simulink model "equalizer_model_deluxe"  (R2014a)
settings: Solver=ode45  StartTime=0.0  StopTime=inf  RelTol=1e-3
libraries: dsparch4 x15, dspmtrx3 x2, dspvision x1, dspobslib x1, dspsrcs4 x1, dspsnks4 x1, dspsigops x1
settings Model: Creator=salvat06  LastModifiedBy=salvat06
settings DebuggingCC: MergeDetectMultiDrivingBlocksExec=error

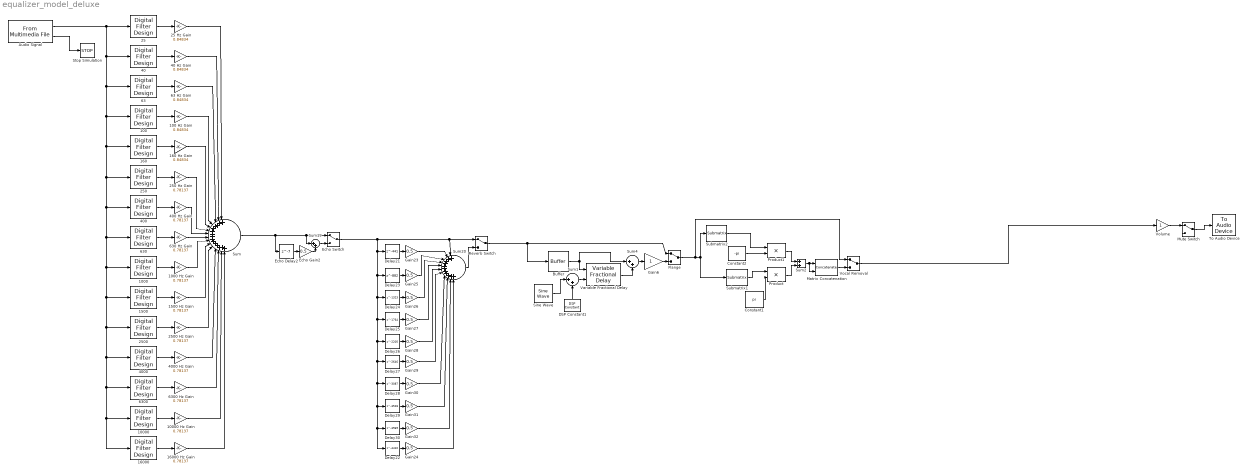
== system equalizer_model_deluxe ==
  {63,100,160,250,400,630,1000,1500,2500,4000,6300,10000,16000} (13 alike) : dsparch4/Digital Filter Design  mwdsp_browser_bugfix_var=off
  100 Hz Gain : Gain  Gain=0.84834
  1000 Hz Gain : Gain  Gain=0.78137
  10000 Hz Gain : Gain  Gain=0.78137
  1500 Hz Gain : Gain  Gain=0.78137
  160 Hz Gain : Gain  Gain=0.84834
  16000 Hz Gain : Gain  Gain=0.78137
  "25 " : dsparch4/Digital Filter Design  mwdsp_browser_bugfix_var=off
  25 Hz Gain : Gain  Gain=0.84834
  250 Hz Gain : Gain  Gain=0.78137
  2500 Hz Gain : Gain  Gain=0.78137
  "40 " : dsparch4/Digital Filter Design  mwdsp_browser_bugfix_var=off
  40 Hz Gain : Gain  Gain=0.84834
  400 Hz Gain : Gain  Gain=0.78137
  4000 Hz Gain : Gain  Gain=0.78137
  63 Hz Gain : Gain  Gain=0.84834
  630 Hz Gain : Gain  Gain=0.78137
  6300 Hz Gain : Gain  Gain=0.78137
  Audio Signal : dspvision/From Multimedia File  inputFilename=\\rowanads.rowan.edu\home\salvat06\documents\A-DSP, Round 2\McCall\James Music Selection\Iron Jaw Gulch.wav  loop=on  numPlays=1  outputStreams=Audio only  videoDataType=single  audioDataType=double  inheritSampleTime=on  userDefinedSampleTime=1/30  noAudioOutput=off  isIntensityVideo=off  fourcc=RGB  colorVideoFormat=Separate color signals  outputEOF=on  dataOrg=Column-major  audioFrameSize=256  computeAudioFrameSize=off  outSamplingMode=Frame based
  Buffer : Buffer  N=256  ic=100
  Constant1 : Constant  Value=pi
  Constant2 : Constant  Value=-pi
  DSP Constant1 : dspobslib/DSP Constant  Value=30  SampleMode=Discrete  discreteOutput=Sample-based (interpret vectors as 1-D)  continuousOutput=Sample-based (interpret vectors as 1-D)  sampTime=256/44100  framePeriod=256/44100  dataType=Inherit from 'Constant value'  isSigned=on  wordLen=16  udDataType=sfix(16)  fracBitsMode=Best precision  numFracBits=15  InterpretAs1D=on  Ts=256/44100  FramebasedOutput=off
  Delay21 : Delay  DelayLength=441  InitialCondition=0  InputProcessing=Inherited
  Delay22 : Delay  DelayLength=4410  InitialCondition=0  InputProcessing=Inherited
  Delay23 : Delay  DelayLength=882  InitialCondition=0  InputProcessing=Inherited
  Delay24 : Delay  DelayLength=1323  InitialCondition=0  InputProcessing=Inherited
  Delay25 : Delay  DelayLength=1764  InitialCondition=0  InputProcessing=Inherited
  Delay26 : Delay  DelayLength=2205  InitialCondition=0  InputProcessing=Inherited
  Delay27 : Delay  DelayLength=2646  InitialCondition=0  InputProcessing=Inherited
  Delay28 : Delay  DelayLength=3087  InitialCondition=0  InputProcessing=Inherited
  Delay29 : Delay  DelayLength=3528  InitialCondition=0  InputProcessing=Inherited
  Delay30 : Delay  DelayLength=3969  InitialCondition=0  InputProcessing=Inherited
  Echo Gain2 : Gain  Gain=0.5
  Echo Delay2 : Delay  DelayLength=7  InitialCondition=0  InputProcessing=Inherited
  Echo Switch : ManualSwitch
  Flange : ManualSwitch
  Gain{23..32} (10 alike) : Gain  Gain=0.5
  Gain6 : Gain  SaturateOnIntegerOverflow=on  OutDataTypeStr=Inherit: Same as input  ParamDataTypeStr=Inherit: Same as input
  Matrix Concatenation : Concatenate  Mode=Multidimensional array  ConcatenateDimension=2
  Mute Switch : ManualSwitch
  Product : Product  SaturateOnIntegerOverflow=on  OutDataTypeStr=Inherit: Same as first input
  Product1 : Product  SaturateOnIntegerOverflow=on  OutDataTypeStr=Inherit: Same as first input
  Reverb Switch : ManualSwitch
  Sine Wave : dspsrcs4/Sine Wave  Amplitude=30  Frequency=1/3.934 * 1.5  Phase=[-pi/4 pi/4]  SampleMode=Discrete  OutComplex=Real  CompMethod=Trigonometric fcn  TableSize=Speed  SampleTime=1/44100  SamplesPerFrame=256  ResetState=Restart at time zero  dataType=double  wordLen=16  udDataType=sfix(16)  fracBitsMode=User-defined  numFracBits=14  OutDataTypeStr=double  LastOutDataTypeStr=double
  Stop Simulation : Stop
  Submatrix1 : dspmtrx3/Submatrix  RowSpan=Range of rows  RowStartMode=First  RowStartIndex=1  RowEndMode=Last  RowEndIndex=1  ColSpan=One column  ColStartMode=Last  ColStartIndex=1  ColEndMode=Last  ColEndIndex=1
  Submatrix2 : dspmtrx3/Submatrix  RowSpan=Range of rows  RowStartMode=First  RowStartIndex=1  RowEndMode=Last  RowEndIndex=1  ColSpan=One column  ColStartMode=First  ColStartIndex=1  ColEndMode=Last  ColEndIndex=1
  Sum : Sum  Inputs=|+++++++++++++++  AccumDataTypeStr=double  OutDataTypeStr=double
  Sum1 : Sum  Inputs=|++  SaturateOnIntegerOverflow=on  InputSameDT=on  OutDataTypeStr=Inherit: Same as first input
  Sum19 : Sum  Inputs=|++
  Sum2 : Sum  SaturateOnIntegerOverflow=on
  Sum20 : Sum  Inputs=|+++++++++++
  Sum4 : Sum  Inputs=|++  SaturateOnIntegerOverflow=on  InputSameDT=on  OutDataTypeStr=Inherit: Same as first input
  To Audio Device : dspsnks4/To Audio Device  deviceName=Default  inheritSampleRate=off  sampleRate=44100  deviceDatatype=Determine from input data type  autoBufferSize=on  bufferSize=4096  queueDuration=1.0  defaultOutputChannelMapping=on  outputChannelMapping=1:2
  Variable Fractional Delay : dspsigops/Variable Fractional Delay  mode=OBSOLETE  modeActive=FIR  dmax=44100*10e-3  InputProcessing=Inherited (this choice will be removed - see release notes)  L=8  FarrowL=4  R=10  alpha=0.5  ic=0  fallbackFIR=Switch to linear interpolation if kernel cannot be centered  fallbackFarrow=Clip to the minimum value necessary for centered kernel  noDFT=off  roundingMode=Zero  overflowMode=off
  Vocal Removal : ManualSwitch
  Volume : Gain  Tag=Volume
  wires:
  "25 "/1 -> 25 Hz Gain/1
  "40 "/1 -> 40 Hz Gain/1
  63/1 -> 63 Hz Gain/1
  100/1 -> 100 Hz Gain/1
  160/1 -> 160 Hz Gain/1
  250/1 -> 250 Hz Gain/1
  400/1 -> 400 Hz Gain/1
  630/1 -> 630 Hz Gain/1
  1000/1 -> 1000 Hz Gain/1
  1500/1 -> 1500 Hz Gain/1
  2500/1 -> 2500 Hz Gain/1
  4000/1 -> 4000 Hz Gain/1
  6300/1 -> 6300 Hz Gain/1
  10000/1 -> 10000 Hz Gain/1
  16000/1 -> 16000 Hz Gain/1
  Audio Signal/2 -> Stop Simulation/1
  Vocal Removal/1 -> Volume/1
  Audio Signal/1 -> "25 "/1, "40 "/1, 63/1, 100/1, 160/1, 250/1, 400/1, 630/1, 1000/1, 1500/1, 4000/1, 6300/1, 10000/1, 16000/1, 2500/1
  25 Hz Gain/1 -> Sum/1
  40 Hz Gain/1 -> Sum/2
  63 Hz Gain/1 -> Sum/3
  100 Hz Gain/1 -> Sum/4
  250 Hz Gain/1 -> Sum/6
  160 Hz Gain/1 -> Sum/5
  400 Hz Gain/1 -> Sum/7
  630 Hz Gain/1 -> Sum/8
  1000 Hz Gain/1 -> Sum/9
  1500 Hz Gain/1 -> Sum/10
  2500 Hz Gain/1 -> Sum/11
  4000 Hz Gain/1 -> Sum/12
  6300 Hz Gain/1 -> Sum/13
  10000 Hz Gain/1 -> Sum/14
  16000 Hz Gain/1 -> Sum/15
  Volume/1 -> Mute Switch/1
  Mute Switch/1 -> To Audio Device/1
  Variable Fractional Delay/1 -> Sum4/2
  Sum4/1 -> Gain6/1
  DSP Constant1/1 -> Sum1/2
  Sine Wave/1 -> Sum1/1
  Sum1/1 -> Variable Fractional Delay/2
  Buffer/1 -> Variable Fractional Delay/1, Sum4/1
  Reverb Switch/1 -> Flange/1, Buffer/1
  Gain6/1 -> Flange/2
  Flange/1 -> Vocal Removal/1, Submatrix2/1, Submatrix1/1
  Submatrix1/1 -> Product/1
  Constant1/1 -> Product/2
  Submatrix2/1 -> Product1/1
  Constant2/1 -> Product1/2
  Product1/1 -> Sum2/1
  Product/1 -> Sum2/2
  Sum2/1 -> Matrix Concatenation/1, Matrix Concatenation/2
  Matrix Concatenation/1 -> Vocal Removal/2
  Echo Delay2/1 -> Echo Gain2/1
  Echo Gain2/1 -> Sum19/2
  Sum19/1 -> Echo Switch/2
  Sum/1 -> Echo Delay2/1, Sum19/1, Echo Switch/1
  Sum20/1 -> Reverb Switch/2
  Delay21/1 -> Gain23/1
  Echo Switch/1 -> Reverb Switch/1, Sum20/1, Delay22/1, Delay30/1, Delay29/1, Delay28/1, Delay27/1, Delay26/1, Delay25/1, Delay24/1, Delay23/1, Delay21/1
  Delay23/1 -> Gain25/1
  Delay24/1 -> Gain26/1
  Delay25/1 -> Gain27/1
  Delay26/1 -> Gain28/1
  Delay27/1 -> Gain29/1
  Delay28/1 -> Gain30/1
  Delay29/1 -> Gain31/1
  Delay30/1 -> Gain32/1
  Delay22/1 -> Gain24/1
  Gain23/1 -> Sum20/2
  Gain25/1 -> Sum20/3
  Gain26/1 -> Sum20/4
  Gain27/1 -> Sum20/5
  Gain28/1 -> Sum20/6
  Gain29/1 -> Sum20/7
  Gain30/1 -> Sum20/8
  Gain31/1 -> Sum20/9
  Gain32/1 -> Sum20/10
  Gain24/1 -> Sum20/11
